simulink model "SpeedgoatCANOpen03"  (R2018b)
settings: Solver=FixedStepDiscrete  StartTime=0.0  StopTime=inf  FixedStep=0.001  RelTol=1e-3  EnableMultiTasking=on
libraries: speedgoatlib_IO691 x6, slrtlib x6
settings Model: SimulationMode=external  Creator=Venqo  LastModifiedBy=Venqo
settings SolverCC: ConcurrentTasks=on  AutoInsertRateTranBlk=on
settings DataIOCC: SaveFormat=StructureWithTime
settings OptimizationCC: BlockReduction=off  OptimizeBlockIOStorage=off  BufferReuse=off  GlobalBufferReuse=off  ExpressionFolding=off  LocalBlockOutputs=off  OptimizeDataStoreBuffers=off  BusAssignmentInplaceUpdate=off
settings HardwareCC: ProdBitPerPointer=32  ProdBitPerSizeT=32  ProdBitPerPtrDiffT=32  ProdLargestAtomicFloat=None  ProdWordSize=32  ProdLongLongMode=on  ProdHWDeviceType=Generic->32-bit x86 compatible
settings SFSimCC: SimCustomHeaderCode="#include \"CANOpenSlave.h\""  SimCustomInitializer=CANOpenSlave_ResetCommunication();  SimUserSources=CANOpenSlave.c
settings RTWCC: SystemTargetFile=slrt.tlc  TemplateMakefile=slrt_default_tmf  Description=Simulink Real-Time  RTWUseSimCustomCode=on  CustomHeaderCode="#include \"CANOpenSlave.h\""  CustomSource=CANOpenSlave.c  CustomInitializer=CANOpenSlave_ResetCommunication();  CodeExecutionProfiling=on  RTWCompilerOptimization=on
settings SimulinkRealTimeCC: InferredTypesCompatibility=on  SupportVariableSizeSignals=on  PreserveStateflowLocalDataDimensions=off  RL32LogTETModifier=off  xPCConcurrentTasks=on

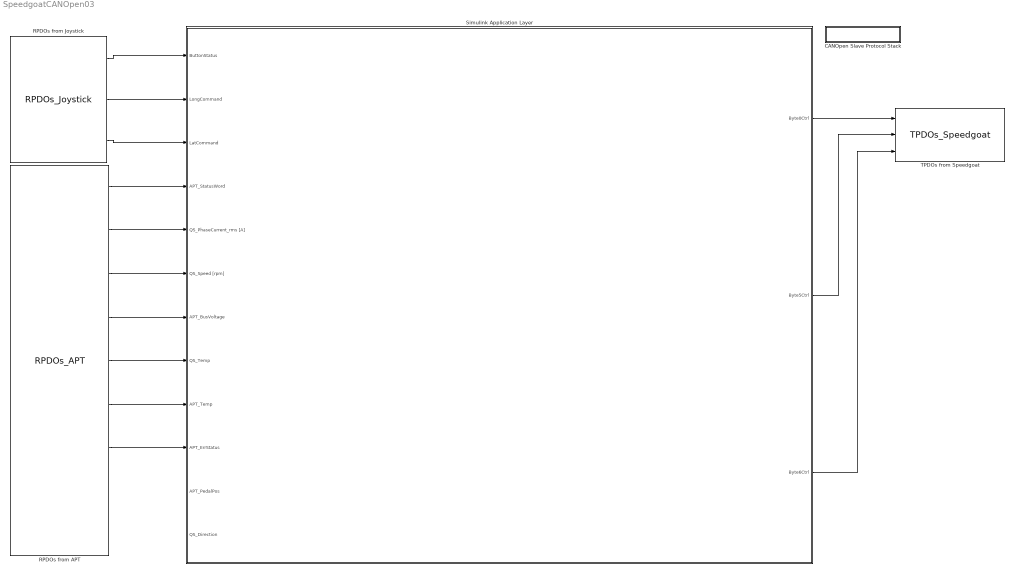
== system SpeedgoatCANOpen03 ==
  CANOpen Slave Protocol Stack : Subsystem  mask{Ts=0.001}
      mask prompts: Ts "Sample Time (s)"
      mask Display: disp('CANOpen Slave Stack')
  RPDOs from APT : S-Function  InitFcn=try, set_param(gcb,'FunctionName','RPDOs_APT'), end  FunctionName=RPDOs_APT  SFunctionModules=RPDOs_APT_wrapper  SFunctionDeploymentMode=off  EnableBusSupport=off  mask(S-Function Builder){}
      mask help: Simulink:masks:SFunctionBuilder_MD
      mask init:
      | val = [[.9  0.75 0.75 1 1 .9 .9 1]',[1 1 0.75 0.75 .9 .9 1 .9]'];try , sys = get_param(gcb,'SfunBuilderFcnName');if isempty(sys), sys = get_param(gcb,'FunctionName'); end,catch, sys = get_param(gcb,'FunctionName'); end
      settings: CopyFcn=set_param(gcbh,'LinkStatus','none')  PreSaveFcn=try, set_param(gcb,'FunctionName','RPDOs_APT'), end  OpenFcn=sfunctionwizard(gcbh)
      mask Display: plot(val(:,1),val(:,2)),disp(sys), port_label('output',1,'StatusWord'), port_label('output',2,'PhaseCurrent'), port_label('output',3,'Speed'), port_label('output',4,'BusVoltage'), port_label('output',5,'MotorTemp'), port_label('output',6,'APTTemp'), port_label('output',7,'ErrStatus'), port_label('output',8,'PedalPos'), port_label('output',9,'Direction')
  RPDOs from Joystick : S-Function  InitFcn=try, set_param(gcb,'FunctionName','RPDOs_Joystick'), end  FunctionName=RPDOs_Joystick  SFunctionModules=RPDOs_Joystick_wrapper  SFunctionDeploymentMode=off  EnableBusSupport=off  mask(S-Function Builder){}
      mask help: Simulink:masks:SFunctionBuilder_MD
      mask init: same as SpeedgoatCANOpen03/RPDOs from APT
      settings: CopyFcn=set_param(gcbh,'LinkStatus','none')  PreSaveFcn=try, set_param(gcb,'FunctionName','RPDOs_Joystick'), end  OpenFcn=sfunctionwizard(gcbh)
      mask Display: plot(val(:,1),val(:,2)),disp(sys), port_label('output',1,'ButtonsStatus'), port_label('output',2,'LongCmd'), port_label('output',3,'LatCmd')
  Simulink Application Layer : Subsystem
  TPDOs from Speedgoat : S-Function  InitFcn=try, set_param(gcb,'FunctionName','TPDOs_Speedgoat'), end  FunctionName=TPDOs_Speedgoat  SFunctionModules=TPDOs_Speedgoat_wrapper  SFunctionDeploymentMode=off  EnableBusSupport=off  mask(S-Function Builder){}
      mask help: Simulink:masks:SFunctionBuilder_MD
      mask init: same as SpeedgoatCANOpen03/RPDOs from APT
      settings: CopyFcn=set_param(gcbh,'LinkStatus','none')  PreSaveFcn=try, set_param(gcb,'FunctionName','TPDOs_Speedgoat'), end  OpenFcn=sfunctionwizard(gcbh)
      mask Display: plot(val(:,1),val(:,2)),disp(sys), port_label('input',1,'Byte0Ctrl'), port_label('input',2,'Byte5Ctrl'), port_label('input',3,'Byte6Ctrl')
  wires:
  RPDOs from Joystick/1 -> Simulink Application Layer/1(ButtonStatus)
  RPDOs from Joystick/2 -> Simulink Application Layer/2(LongCommand)
  RPDOs from Joystick/3 -> Simulink Application Layer/3(LatCommand)
  Simulink Application Layer/1(Byte0Ctrl) -> TPDOs from Speedgoat/1
  Simulink Application Layer/2(Byte5Ctrl) -> TPDOs from Speedgoat/2
  Simulink Application Layer/3(Byte6Ctrl) -> TPDOs from Speedgoat/3
  RPDOs from APT/3 -> Simulink Application Layer/6(QS_Speed [rpm])
  RPDOs from APT/1 -> Simulink Application Layer/4(APT_StatusWord)
  RPDOs from APT/2 -> Simulink Application Layer/5(QS_PhaseCurrent_rms [A])
  RPDOs from APT/4 -> Simulink Application Layer/7(APT_BusVoltage)
  RPDOs from APT/5 -> Simulink Application Layer/8(QS_Temp)
  RPDOs from APT/6 -> Simulink Application Layer/9(APT_Temp)
  RPDOs from APT/7 -> Simulink Application Layer/10(APT_ErrStatus)
  ? -> Simulink Application Layer/12(QS_Direction)

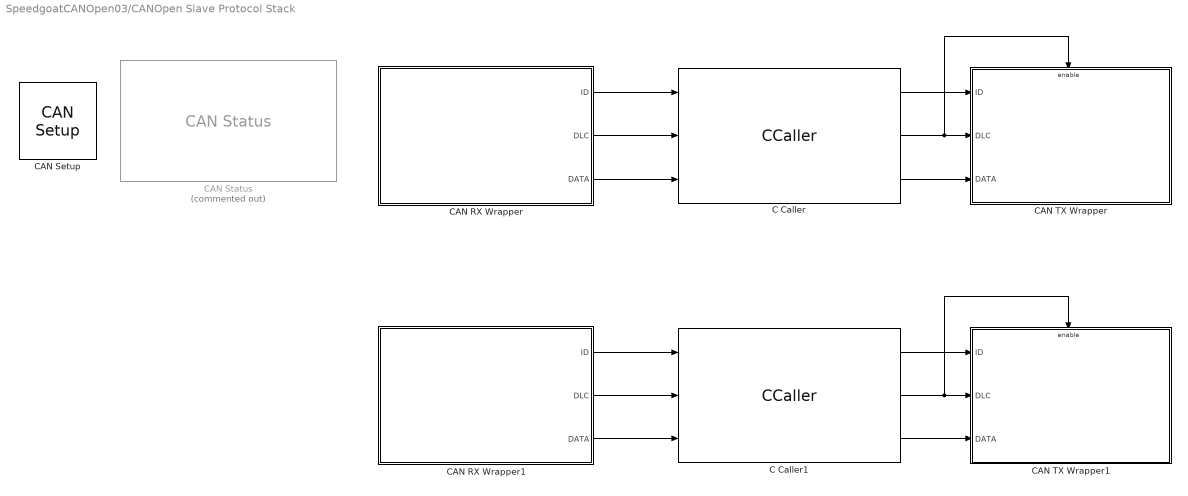
== system SpeedgoatCANOpen03/CANOpen Slave Protocol Stack ==
  C Caller : CCaller  FunctionName=CANOpenSlave_ProcessStack  PortSpecificationStruct="%)30     .    ( D   8    (     @         %    \"     8    !     0         %  0 \"0    $    V    07)G3F%M90  4&]R=$YA;64 4V-O<&4     26YD97@     5'EP90      4VEZ90         .    ,     8    (    !          %    \"     $    $     0         0  0 <GA)1 X    P    !@    @    $          4    (     0    0    !         !  ! !R>$E$#@   #@    &    \"     0         !0    @    !    !0    $         $     4   !);G ...(+2763 chars)"
  C Caller1 : CCaller  FunctionName=CANOpenSlave_ProcessStack  PortSpecificationStruct="%)30     .    ( D   8    (     @         %    \"     8    !     0         %  0 \"0    $    V    07)G3F%M90  4&]R=$YA;64 4V-O<&4     26YD97@     5'EP90      4VEZ90         .    ,     8    (    !          %    \"     $    $     0         0  0 <GA)1 X    P    !@    @    $          4    (     0    0    !         !  ! !R>$E$#@   #@    &    \"     0         !0    @    !    !0    $         $     4   !);G ...(+2763 chars)"
  CAN RX Wrapper : Subsystem
  CAN RX Wrapper1 : Subsystem
  "CAN Setup " : speedgoatlib_IO691/CAN Setup   moduletype=IO691  id=1  pciSlot=-1  chn1=CAN (HS)  chn2=CAN (HS)  chn3=Disabled  chn4=Disabled  initStruct=[]  termStruct=[]  ArbitrationbdrChn1=500 kBaud  ArbitrationManbdrChn1=[2,16,63,16]  FdbdrChn1=5.0 MBaud  FdManbdrChn1=[2,2,5,2]  ArbitrationbdrChn2=500 kBaud  ArbitrationManbdrChn2=[2,16,63,16]  FdbdrChn2=5.0 MBaud  FdManbdrChn2=[2,2,5,2]  ArbitrationbdrChn3=1.0 MBaud  ArbitrationManbdrChn3=[2,8,31,8]  FdbdrChn3=5.0 MBaud  FdManbdrChn3=[2,2,5,2]  ArbitrationbdrChn4=1.0 MBaud  ArbitrationManbdrChn4=[2,8,31,8]  FdbdrChn4=5.0 MBaud  FdManbdrChn4=[2,2,5,2]  moduleInitValues=[691 1 -1 -1]
      settings: SourceProductName=Simulink Real-Time: Speedgoat Library
  CAN Status : speedgoatlib_IO691/CAN Status  Commented=on  moduleId=1  sampleTime=Ts  channel=1  busRecovery=Off  arrayOutput=off  controllerCpuLoad=off  controllerLiveCount=off  initModeAct=on  avgBusLoad=off  receiving=off  RxQueueEmpty=on  dataOverrunRcv=on  rxBufferLevel=off  txPending=off  dataOverrunTx=on  txBufferLevel=off  errWarnLimit=off  errPassLimit=off  errBusOff=off  busRecoveryCounter=off  busCouplingErr=off  transceiverErr=off  opMode=off  brp=off  timeSegment1=off  timeSegment2=off  synchronisationJumpWidth=off  dataTSEG1=off  dataTSEG2=off  dataSJW=off  moduleType=691  qtyStatBlk=1  ptIdx=0  isFDMod=0
      settings: SourceProductName=Simulink Real-Time: Speedgoat Library
  CAN TX Wrapper : Subsystem
  CAN TX Wrapper1 : Subsystem
  wires:
  C Caller/2 -> CAN TX Wrapper/Enable, CAN TX Wrapper/2(DLC)
  CAN RX Wrapper/1(ID) -> C Caller/1
  C Caller/1 -> CAN TX Wrapper/1(ID)
  CAN RX Wrapper/2(DLC) -> C Caller/2
  C Caller/3 -> CAN TX Wrapper/3(DATA)
  CAN RX Wrapper/3(DATA) -> C Caller/3
  CAN RX Wrapper1/3(DATA) -> C Caller1/3
  C Caller1/3 -> CAN TX Wrapper1/3(DATA)
  CAN RX Wrapper1/2(DLC) -> C Caller1/2
  C Caller1/1 -> CAN TX Wrapper1/1(ID)
  CAN RX Wrapper1/1(ID) -> C Caller1/1
  C Caller1/2 -> CAN TX Wrapper1/2(DLC), CAN TX Wrapper1/Enable

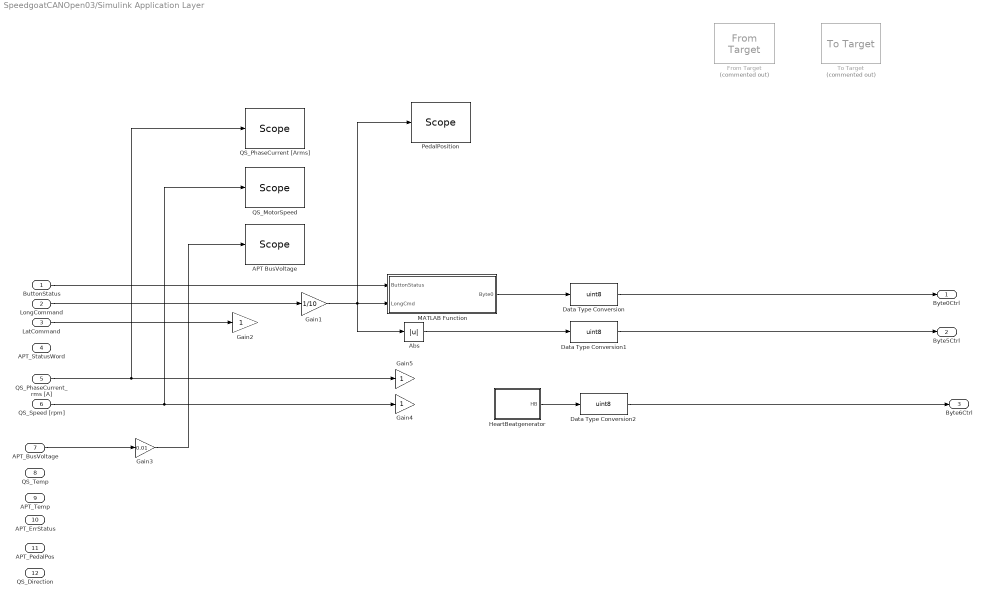
== system SpeedgoatCANOpen03/Simulink Application Layer ==
  ButtonStatus : Inport  OutDataTypeStr=uint8
  LongCommand : Inport  Port=2
  LatCommand : Inport  Port=3
  APT_StatusWord : Inport  Port=4
  QS_PhaseCurrent_rms [A] : Inport  Port=5
  QS_Speed [rpm] : Inport  Port=6  OutDataTypeStr=int16
  APT_BusVoltage : Inport  Port=7
  QS_Temp : Inport  Port=8
  APT_Temp : Inport  Port=9
  APT_ErrStatus : Inport  Port=10
  APT_PedalPos : Inport  Port=11
  QS_Direction : Inport  Port=12
  APT BusVoltage : slrtlib/Displays and Logging/Scope   scopeno=3  scopetype=Target  autostart=on  viewmode=Graphical sliding  formatstr='%15.6f'  grid=on  ylimits=[0,60]  nosamples=25000  noprepostsamples=0  interleave=1  triggermode=FreeRun  triggersignal=1  trigsignalfromport=off  triggerlevel=0.0  triggerslope=Rising  triggerscope=1  triggersample=0  filename=data.dat  mode=Lazy  writesize=512  autorestart=off  dynamicfilemode=off  maxwritefilesize=512*1024^2
  Abs : Abs
  Data Type Conversion : DataTypeConversion  OutDataTypeStr=uint8
  Data Type Conversion1 : DataTypeConversion  OutDataTypeStr=uint8
  Data Type Conversion2 : DataTypeConversion  OutDataTypeStr=uint8
  "From Target " : slrtlib/Displays and Logging/From Target   Commented=on  appname=''  blockpath=block  ts=1  isdefault=on
      settings: SourceProductName=Simulink Real-Time  SourceProductBaseCode=XP
  Gain1 : Gain  Gain=1/10
  Gain2 : Gain
  Gain3 : Gain  Gain=0.01  OutDataTypeStr=single
  Gain4 : Gain  OutDataTypeStr=single
  Gain5 : Gain  OutDataTypeStr=single
  HeartBeatgenerator : MATLAB Function  TreatAsAtomicUnit=on
  MATLAB Function : MATLAB Function  TreatAsAtomicUnit=on
  PedalPosition : slrtlib/Displays and Logging/Scope   scopeno=4  scopetype=Target  autostart=on  viewmode=Graphical sliding  formatstr='%15.6f'  grid=on  ylimits=[-110,110]  nosamples=25000  noprepostsamples=0  interleave=1  triggermode=FreeRun  triggersignal=1  trigsignalfromport=off  triggerlevel=0.0  triggerslope=Rising  triggerscope=1  triggersample=0  filename=data.dat  mode=Lazy  writesize=512  autorestart=off  dynamicfilemode=off  maxwritefilesize=512*1024^2
  "QS_MotorSpeed " : slrtlib/Displays and Logging/Scope   scopeno=2  scopetype=Target  autostart=on  viewmode=Graphical sliding  formatstr='%15.6f'  grid=on  ylimits=[-100,800]  nosamples=25000  noprepostsamples=0  interleave=1  triggermode=FreeRun  triggersignal=1  trigsignalfromport=off  triggerlevel=0.0  triggerslope=Rising  triggerscope=1  triggersample=0  filename=data.dat  mode=Lazy  writesize=512  autorestart=off  dynamicfilemode=off  maxwritefilesize=512*1024^2
  QS_PhaseCurrent [Arms] : slrtlib/Displays and Logging/Scope   scopeno=1  scopetype=Target  autostart=on  viewmode=Graphical sliding  formatstr='%15.6f'  grid=on  ylimits=[-5,10]  nosamples=25000  noprepostsamples=0  interleave=1  triggermode=FreeRun  triggersignal=1  trigsignalfromport=off  triggerlevel=0.0  triggerslope=Rising  triggerscope=1  triggersample=0  filename=data.dat  mode=Lazy  writesize=512  autorestart=off  dynamicfilemode=off  maxwritefilesize=512*1024^2
  "To Target " : slrtlib/Displays and Logging/To Target   Commented=on  appname=''  blockpath=block  paramname=parameter  isdefault=on
      settings: SourceProductName=Simulink Real-Time  SourceProductBaseCode=XP
  Byte0Ctrl : Outport  OutDataTypeStr=uint8
  Byte5Ctrl : Outport  Port=2  OutDataTypeStr=uint8
  Byte6Ctrl : Outport  Port=3  OutDataTypeStr=uint8
  wires:
  LatCommand/1 -> Gain2/1
  ButtonStatus/1 -> MATLAB Function/1(ButtonStatus)
  LongCommand/1 -> Gain1/1
  QS_PhaseCurrent_rms [A]/1 -> QS_PhaseCurrent [Arms]/1, Gain5/1
  QS_Speed [rpm]/1 -> Gain4/1, "QS_MotorSpeed "/1
  APT_BusVoltage/1 -> Gain3/1
  Gain3/1 -> APT BusVoltage/1
  Gain1/1 -> Abs/1, PedalPosition/1, MATLAB Function/2(LongCmd)
  MATLAB Function/1(Byte0) -> Data Type Conversion/1
  Data Type Conversion/1 -> Byte0Ctrl/1
  Abs/1 -> Data Type Conversion1/1
  Data Type Conversion1/1 -> Byte5Ctrl/1
  HeartBeatgenerator/1(HB) -> Data Type Conversion2/1
  Data Type Conversion2/1 -> Byte6Ctrl/1

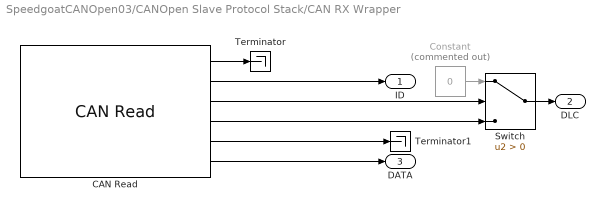
== system SpeedgoatCANOpen03/CANOpen Slave Protocol Stack/CAN RX Wrapper ==
  CAN Read : speedgoatlib_IO691/CAN Read  id=1  ts=Ts  channel=1  messageType=RAW  canType=CAN (HS)  initValues=[691 1 0.001 0 2 1]
      settings: SourceProductName=Simulink Real-Time: Speedgoat Library
  Constant : Constant  Commented=on  Value=0  OutDataTypeStr=Inherit: Inherit via back propagation
  Switch : Switch  Criteria=u2 > Threshold
  Terminator : Terminator
  Terminator1 : Terminator
  ID : Outport
  DLC : Outport  Port=2
  DATA : Outport  Port=3
  wires:
  CAN Read/4 -> Switch/3
  CAN Read/5 -> Terminator1/1
  Switch/1 -> DLC/1
  CAN Read/2 -> ID/1
  CAN Read/3 -> Switch/2
  CAN Read/6 -> DATA/1
  Constant/1 -> Switch/1
  CAN Read/1 -> Terminator/1

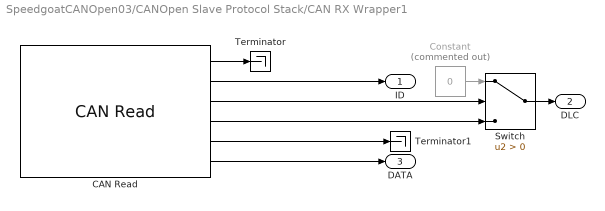
== system SpeedgoatCANOpen03/CANOpen Slave Protocol Stack/CAN RX Wrapper1 ==
  CAN Read : speedgoatlib_IO691/CAN Read  id=1  ts=Ts  channel=2  messageType=RAW  canType=CAN (HS)  initValues=[691 1 0.001 1 2 1]
      settings: SourceProductName=Simulink Real-Time: Speedgoat Library
  Constant : Constant  Commented=on  Value=0  OutDataTypeStr=Inherit: Inherit via back propagation
  Switch : Switch  Criteria=u2 > Threshold
  Terminator : Terminator
  Terminator1 : Terminator
  ID : Outport
  DLC : Outport  Port=2
  DATA : Outport  Port=3
  wires:
  CAN Read/1 -> Terminator/1
  Constant/1 -> Switch/1
  CAN Read/6 -> DATA/1
  CAN Read/3 -> Switch/2
  CAN Read/2 -> ID/1
  Switch/1 -> DLC/1
  CAN Read/5 -> Terminator1/1
  CAN Read/4 -> Switch/3

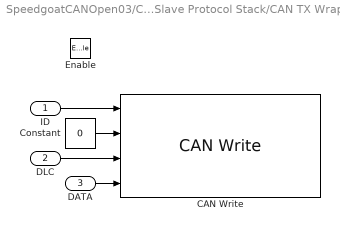
== system SpeedgoatCANOpen03/CANOpen Slave Protocol Stack/CAN TX Wrapper ==
  ID : Inport
  DLC : Inport  Port=2
  DATA : Inport  Port=3
  Enable : EnablePort
  CAN Write : speedgoatlib_IO691/CAN Write  id=1  ts=Ts  channel=1  messageType=RAW  enableStatusPort=off  canType=CAN (HS)  initValues=[691 1 0.001 0 2 1 0]
      settings: SourceProductName=Simulink Real-Time: Speedgoat Library
  Constant : Constant  Value=0  OutDataTypeStr=Inherit: Inherit via back propagation
  wires:
  ID/1 -> CAN Write/1
  DATA/1 -> CAN Write/4
  DLC/1 -> CAN Write/3
  Constant/1 -> CAN Write/2

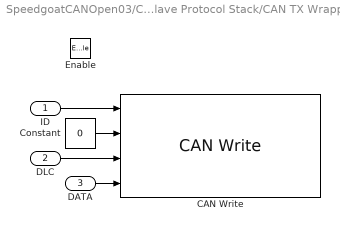
== system SpeedgoatCANOpen03/CANOpen Slave Protocol Stack/CAN TX Wrapper1 ==
  ID : Inport
  DLC : Inport  Port=2
  DATA : Inport  Port=3
  Enable : EnablePort
  CAN Write : speedgoatlib_IO691/CAN Write  id=1  ts=Ts  channel=2  messageType=RAW  enableStatusPort=off  canType=CAN (HS)  initValues=[691 1 0.001 1 2 1 0]
      settings: SourceProductName=Simulink Real-Time: Speedgoat Library
  Constant : Constant  Value=0  OutDataTypeStr=Inherit: Inherit via back propagation
  wires:
  Constant/1 -> CAN Write/2
  DLC/1 -> CAN Write/3
  DATA/1 -> CAN Write/4
  ID/1 -> CAN Write/1

== matlab function SpeedgoatCANOpen03/Simulink Application Layer/HeartBeatgenerator ==
  data: HB output
function HB = HBGenerator
persistent tact Heartbeat
if (isempty(Heartbeat))
    Heartbeat = 0;
    tact = 0;
end
tact=tact+1;
if (tact>10)
    tact=0;
    Heartbeat=Heartbeat+1;
    if (Heartbeat>127)
        Heartbeat = 0;    
    end
end
HB = Heartbeat;

== matlab function SpeedgoatCANOpen03/Simulink Application Layer/MATLAB Function ==
  data: ButtonStatus input; Byte0 output; LongCmd input
function Byte0 = TracCtrl(ButtonStatus, LongCmd)
Direction =0;
if (ButtonStatus>=127)
    if(LongCmd>0)
        Direction = 4;
    elseif (LongCmd<0)
        Direction = 8;
    end
 end
Byte0 =160+Direction;
